simulink model "fm_mod1"  (R2019b)
settings: Solver=VariableStepAuto  StartTime=0.0  StopTime=10.0  RelTol=1e-3
settings Model: Creator=LENOVO  LastModifiedBy=LENOVO

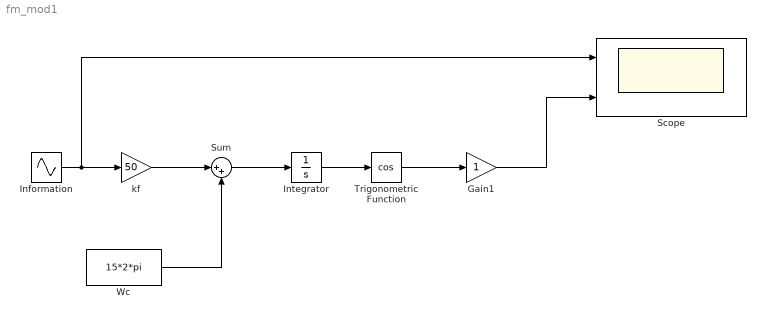
== system fm_mod1 ==
  Gain1 : Gain
  Information : Sin  Frequency=2*pi  SampleTime=0.001
  Integrator : Integrator
  Scope : Scope  NumInputPorts=2
  Sum : Sum  Inputs=|++
  Trigonometric Function : Trigonometry  Operator=cos
  Wc : Constant  Value=15*2*pi
  kf : Gain  Gain=50
  wires:
  kf/1 -> Sum/1
  Wc/1 -> Sum/2
  Sum/1 -> Integrator/1
  Integrator/1 -> Trigonometric Function/1
  Trigonometric Function/1 -> Gain1/1
  Information/1 -> Scope/1, kf/1
  Gain1/1 -> Scope/2
